simulink model "TorqueConv"  (Simulink 6.6)
settings: Solver=ode15s  StartTime=0.0  StopTime=20  MaxStep=0.05  RelTol=1e-3
undefined symbols (not defined in the file or in its folder): accimpeller
settings Model: Creator=Messer  LastModifiedBy=Messer
settings DebuggingCC: SignalResolutionControl=TryResolveAllWithWarning  MultiTaskDSMMsg=warning  MultiTaskCondExecSysMsg=none  StrictBusMsg=None
settings RTWCC: IncludeERTFirstTime=on

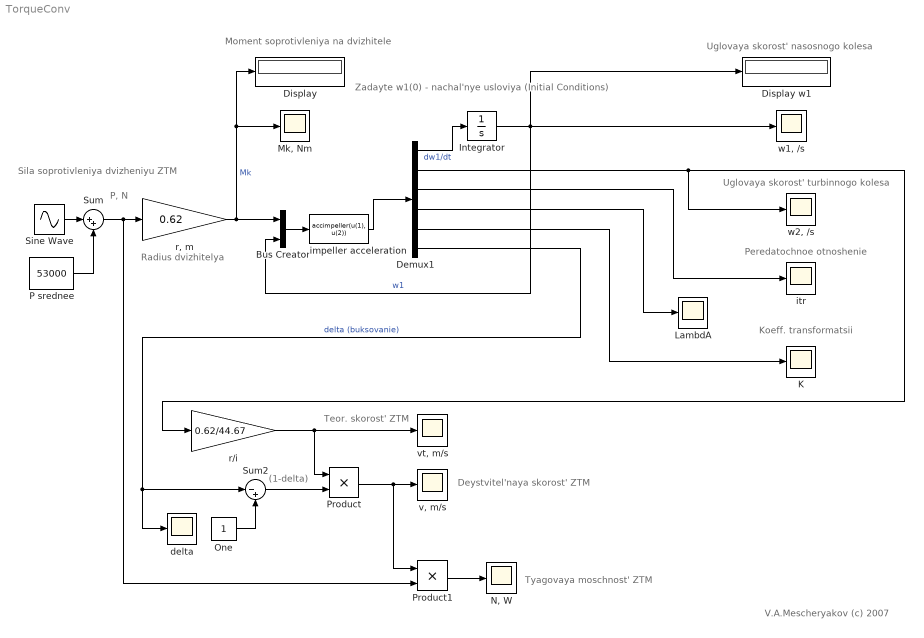
== system TorqueConv ==
  note: P, N
  note: Uglovaya skorost' nasosnogo kolesa
  note: Uglovaya skorost' turbinnogo kolesa
  note: Peredatochnoe otnoshenie
  note: Koeff. transformatsii
  note: Teor. skorost' ZTM
  note: Deystvitel'naya skorost' ZTM
  note: Tyagovaya moschnost' ZTM
  note: Radius dvizhitelya
  note: Moment soprotivleniya na dvizhitele
  note: Sila soprotivleniya
      | dvizheniyu ZTM
  note: (1-delta)
  note: Zadayte w1(0) -
      | nachal'nye usloviya
      | (Initial Conditions)
  note: V.A.Mescheryakov (c) 2007
  Bus Creator : BusCreator  Inputs=2
  Demux1 : Demux  Outputs=6
  Display : Display
  Display w1 : Display
  Integrator : Integrator  InitialCondition=178.5
  K : Scope
      settings: YMin=1.3  YMax=1.55  SaveName=ScopeData7
  LambdA : Scope
      settings: YMin=0.0155  YMax=0.0164  SaveName=ScopeData6
  "Mk, Nm" : Scope
      settings: YMin=30000  YMax=36000
  "N, W" : Scope
      settings: YMin=62000  YMax=67000  SaveName=ScopeData9
  One : Constant
  P srednee : Constant  Value=53000
  Product : Product  RndMeth=Zero
  Product1 : Product  RndMeth=Zero
  Sine Wave : Sin  Amplitude=5000  SampleTime=0
  Sum : Sum  Inputs=|++
  Sum2 : Sum  Inputs=|-+
  delta : Scope
      settings: YMin=0.1  YMax=0.19  SaveName=ScopeData10
  impeller acceleration : MATLABFcn  MATLABFcn=accimpeller(u(1), u(2))  OutputDimensions=6
  itr : Scope
      settings: YMin=0.525  YMax=0.625  SaveName=ScopeData5
  "r, m" : Gain  Gain=0.62
  r/i : Gain  Gain=0.62/44.67
  "v, m/s" : Scope
      settings: YMin=1.05  YMax=1.4  SaveName=ScopeData8
  "vt, m/s" : Scope
      settings: YMin=1.325  YMax=1.55
  "w1, /s" : Scope
      settings: YMin=178.2  YMax=179.1  SaveName=ScopeData2
  "w2, /s" : Scope
      settings: YMin=95  YMax=112.5  SaveName=ScopeData4
  wires:
  "r, m"/1 -> Bus Creator/1, Display/1, "Mk, Nm"/1  "Mk"
  Bus Creator/1 -> impeller acceleration/1
  Integrator/1 -> "w1, /s"/1, Bus Creator/2, Display w1/1  "w1"
  Demux1/2 -> "w2, /s"/1, r/i/1
  Demux1/3 -> itr/1
  Demux1/4 -> LambdA/1
  Demux1/5 -> K/1
  r/i/1 -> "vt, m/s"/1, Product/1
  Product/1 -> "v, m/s"/1, Product1/1
  Product1/1 -> "N, W"/1
  One/1 -> Sum2/2
  Sum2/1 -> Product/2
  Sine Wave/1 -> Sum/1
  P srednee/1 -> Sum/2
  Sum/1 -> "r, m"/1, Product1/2
  Demux1/6 -> Sum2/1, delta/1  "delta (buksovanie)"
  impeller acceleration/1 -> Demux1/1
  Demux1/1 -> Integrator/1  "dw1/dt"
